simulink model "trex"  (Simulink 8.5)
settings: Solver=ode45  SolverMode=SingleTasking  StartTime=0.0  StopTime=0.2  RelTol=1e-3  AbsTol=1e-3
libraries: elements x2, inputs x1
settings Model: Creator=PC  LastModifiedBy=PC
settings DataIOCC: LimitDataPoints=off
settings OptimizationCC: BlockReduction=off  BooleanDataType=off  ExpressionDepthLimit=128
settings DebuggingCC: SaveWithParameterizedLinksMsg=none  SignalResolutionControl=TryResolveAllWithWarning  MultiTaskDSMMsg=warning  MultiTaskCondExecSysMsg=none  FcnCallInpInsideContextMsg=EnableAllAsError  StateNameClashWarn=none  StrictBusMsg=None
settings HardwareCC: TargetUnknown=on
settings RTWCC: TemplateMakefile=grt_vc.tmf

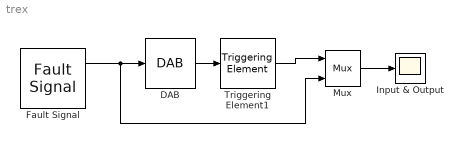
== system trex ==
  DAB : elements/DAB  filter=off  approx=Bessel  order=2  numerator=[]  denominator=[]  freq=200  resdis=on  vertres=12  xmax=5  winsize=20  G=1.0  fs=60*20
  Fault Signal : inputs/Fault Signal  pre_fault=[1 0]  post_fault=[2 90]  fr_dc=[60 0.03 0.0004]  oscA=[1.0 0.8 0.9]  oscf=[1000 3000 8000]  oscT=[ 0.050 0.030 0.060]
  Input & Output : Scope
      settings: TickLabels=on  YMin=-3.5  YMax=3.5
  Mux : Mux  Inputs=2
  Triggering Element1 : elements/Triggering Element  METHOD=Cycle to cycle  TH=.5  p=2  q=5  SF=60*20  SN=20  ti=0.02
  wires:
  DAB/1 -> Triggering Element1/1
  Mux/1 -> Input & Output/1
  Triggering Element1/1 -> Mux/1
  Fault Signal/1 -> Mux/2, DAB/1
